simulink model "unittest"  (R2020b)
settings: Solver=VariableStepAuto  StartTime=0.0  StopTime=5  RelTol=1e-3
settings Model: Creator=mateu  LastModifiedBy=mateu

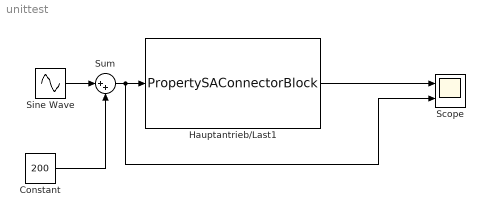
== system unittest ==
  Constant : Constant  Value=200
  Hauptantrieb/Last1 : S-Function  FunctionName=PropertySAConnectorBlock  Parameters=bm, sr, regUrlStr, aasUrlStr, aasId, smId, seId  SFunctionDeploymentMode=off  EnableBusSupport=off  mask{bmStr=Snapshot, conMethod=via RegistryServer, aasUrlStr_=http://localhost:4001/aasServer/shells/https%3A%2F%2Fexample.com%2Fids%2Faas%2F6001_2130_8022_6165/aas, regUrlStr=http://localhost:8082/registry/api/v1/registryasd, sr=0.1, aasId=https://example.com/ids/aas/6001_2130_8022_6165, smId=Hauptantrieb, seId=last, bm=0, aasUrlStr=}
      mask prompts: bmStr "Operation Mode"; conMethod "Connection Method"; aasUrlStr_ "AAS Url"; regUrlStr "Registry URL"; sr "Sample Rate"; aasId "AAS Id"; smId "Submodel IdShort"; seId "Property IdShort"
      mask TypeOptions bmStr: Snapshot | Real-time
      mask Callback bmStr:
      | bmStr = get_param(gcb,'bmStr');
      | vis = get_param(gcb,'MaskVisibilities');
      | 
      | switch bmStr
      |     case 'Snapshot'
      |         set_param(gcb, 'bm', "0");
      |         vis(5) = {'off'};
      |         set_param(gcb, 'MaskVisibilities', vis);
      |     case 'Real-time'
      |         set_param(gcb, 'bm',  "1");
      |         vis(5) = {'on'};
      |         set_param(gcb, 'MaskVisibilities', vis);
      | end
      mask TypeOptions conMethod: via RegistryServer | via AAS URL
      mask Callback conMethod:
      | conMethod = get_param(gcb,'conMethod');
      | aasUrlStr = get_param(gcb,'aasUrlStr_');
      | vis = get_param(gcb,'MaskVisibilities');
      | 
      | switch conMethod
      |     case 'via RegistryServer'
      |         vis(3) = {'off'};
      |         vis(4) = {'on'};
      |         set_param(gcb, 'MaskVisibilities', vis);
      |         set_param(gcb, 'aasUrlStr', '');
      |     case 'via AAS URL'
      |         vis(3) = {'on'};
      |         vis(4) = {'off'};
      |         set_param(gcb, 'MaskVisibilities', vis);
      |         set_param(gcb, 'aasUrlStr', aasUrlStr);
      | end
      mask Callback aasUrlStr_:
      | conMethod = get_param(gcb,'conMethod');
      | aasUrlStr = get_param(gcb,'aasUrlStr_');
      | switch conMethod
      |     case 'via AAS URL'
      |         set_param(gcb, 'aasUrlStr', aasUrlStr);
      | end
      mask DialogControl DescGroupVar Prompt: Standalone Property Block
      mask DialogControl DescTextVar Prompt: This block connects to a SubmodelElement running in an AAS Server. Data sent to the block's input updates the value of the SubmodelElement, whereas its current value is sent to the block's output. This process can be executed in two operation modes: Snapshot mode, wherein the input routine is executed at the beginining and the output routine at the end of the simulation; Real-time mode, by which is assumed that the wall clock is the same as the simulation clock and the input/output routines are executed in the specified sample rate.
      mask Display:
      | bm = get_param(gcb,'bm')
      | sr = get_param(gcb,'sr')
      | aas = replace(get_param(gcb,'aasId'),"_","\_");
      | sm = replace(get_param(gcb,'smId'),"_","\_");
      | se = replace(get_param(gcb,'seId'),"_","\_");
      | 
      | pos = get_param(gcb, 'Position');
      | w = pos(3) - pos(1);
      | h = pos(4) - pos(2);
      | 
      | full = sm  + "/" + se
      | text(5,20, "{\bf\fontsize{7}"+aas+"}", 'texmode','on')
      | text(5,10, "{\bf\fontsize{6}"+full+"}", 'texmode','on')
      | image('basyx.png', [w-15,h-20,10,15]);
      | 
      | if bm=="1"
      |     port_label('output', 1,"{\bf\fontsize{6}sr="+sr+"s}", 'texmode','on')
      | end
  Scope : Scope  NumInputPorts=2
  Sine Wave : Sin  Amplitude=50  SampleTime=0
  Sum : Sum  Inputs=|++
  wires:
  Sine Wave/1 -> Sum/1
  Sum/1 -> Scope/2, Hauptantrieb/Last1/1
  Constant/1 -> Sum/2
  Hauptantrieb/Last1/1 -> Scope/1
